simulink model "hdl_top_level_simulation"  (R2017b)
settings: Solver=VariableStepAuto  StartTime=0.0  StopTime=2  RelTol=1e-3
libraries: commchan3 x1, simulink x1
settings Model: Creator=jake  LastModifiedBy=mw
settings CodeAppCC: StateflowObjectComments=on

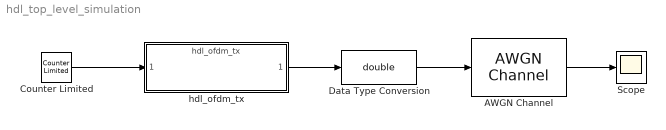
== system hdl_top_level_simulation ==
  AWGN Channel : commchan3/AWGN Channel  InputProcessing=Columns as channels (frame based)  seed=67  noiseMode="Signal to noise ratio  (Eb/No)"  EbNodB=10  EsNodB=10  SNRdB=10  bitsPerSym=1  Ps=1  Tsym=1  variance=1
  Counter Limited : simulink/Sources/Counter Limited  uplimit=14  tsamp=-1
  Data Type Conversion : DataTypeConversion  OutDataTypeStr=double
  Scope : Scope
  hdl_ofdm_tx : ModelReference  ModelNameDialog=hdl_ofdm_tx.slx  SimulationMode=Normal  ModelReferenceVersion=1.38
  wires:
  Counter Limited/1 -> hdl_ofdm_tx/1
  hdl_ofdm_tx/1 -> Data Type Conversion/1
  AWGN Channel/1 -> Scope/1
  Data Type Conversion/1 -> AWGN Channel/1
